simulink library "GPS_processing_lib"  (R2016b)
settings: Solver=VariableStepAuto  StartTime=0.0  StopTime=10.0  RelTol=1e-3
undefined symbols (not defined in the file or in its folder): fsw_params
libraries: time_conversion_lib x1, ecef_2_TLE_lib x1
settings Model: Creator=taylorreynolds  LastModifiedBy=taylorreynolds

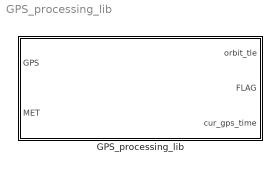
== system GPS_processing_lib ==
  GPS_processing_lib : Subsystem

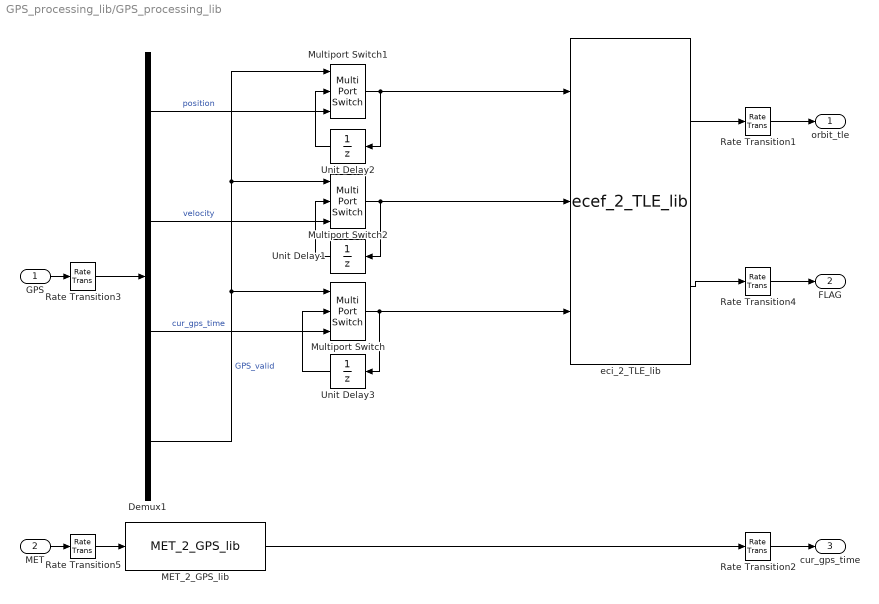
== system GPS_processing_lib/GPS_processing_lib ==
  GPS : Inport
  MET : Inport  Port=2
  Demux1 : Demux  Outputs=[3 3 2 1]
  MET_2_GPS_lib : time_conversion_lib/MET_2_GPS_lib
  Multiport Switch : MultiPortSwitch  DataPortOrder=Zero-based contiguous  Inputs=2
  Multiport Switch1 : MultiPortSwitch  DataPortOrder=Zero-based contiguous  Inputs=2
  Multiport Switch2 : MultiPortSwitch  DataPortOrder=Zero-based contiguous  Inputs=2
  Rate Transition1 : RateTransition  X0=fsw_params.bus.orbit_tle
  Rate Transition2 : RateTransition  Deterministic=off  X0=fsw_params.sensor_processing.gps.ic.time
  Rate Transition3 : RateTransition  X0=fsw_params.sensor_processing.gps.ic.all  OutPortSampleTime=fsw_params.sensor_processing.gps.sample_time_s
  Rate Transition4 : RateTransition
  Rate Transition5 : RateTransition  X0=fsw_params.sensor_processing.gps.JD_J2000_TT_s  OutPortSampleTime=fsw_params.sensor_processing.gps.sample_time_s
  Unit Delay1 : UnitDelay  InitialCondition=fsw_params.sensor_processing.gps.ic.vel_ecef_mps  SampleTime=-1
  Unit Delay2 : UnitDelay  InitialCondition=fsw_params.sensor_processing.gps.ic.pos_ecef_m  SampleTime=-1
  Unit Delay3 : UnitDelay  InitialCondition=fsw_params.sensor_processing.gps.ic.time  SampleTime=-1
  eci_2_TLE_lib : ecef_2_TLE_lib/ecef_2_TLE_lib
  orbit_tle : Outport
  FLAG : Outport  Port=2
  cur_gps_time : Outport  Port=3
  wires:
  MET_2_GPS_lib/1 -> Rate Transition2/1
  Rate Transition5/1 -> MET_2_GPS_lib/1
  MET/1 -> Rate Transition5/1
  Unit Delay3/1 -> Multiport Switch/2
  Multiport Switch/1 -> Unit Delay3/1, eci_2_TLE_lib/3
  eci_2_TLE_lib/2 -> Rate Transition4/1
  Rate Transition4/1 -> FLAG/1
  Rate Transition3/1 -> Demux1/1
  Rate Transition1/1 -> orbit_tle/1
  Rate Transition2/1 -> cur_gps_time/1
  Demux1/4 -> Multiport Switch/1, Multiport Switch1/1, Multiport Switch2/1  "GPS_valid"
  Demux1/3 -> Multiport Switch/3  "cur_gps_time"
  eci_2_TLE_lib/1 -> Rate Transition1/1
  Demux1/2 -> Multiport Switch2/3  "velocity"
  Demux1/1 -> Multiport Switch1/3  "position"
  GPS/1 -> Rate Transition3/1
  Unit Delay1/1 -> Multiport Switch2/2
  Unit Delay2/1 -> Multiport Switch1/2
  Multiport Switch1/1 -> Unit Delay2/1, eci_2_TLE_lib/1
  Multiport Switch2/1 -> Unit Delay1/1, eci_2_TLE_lib/2
